simulink model "Galvo_sys_v1"  (R2013a)
settings: Solver=ode45  StartTime=0.0  StopTime=SimEnd  MaxStep=1e-7  RelTol=1e-3
PreLoadFcn:
  | SimEnd = evalin('base','SimEnd');
  | Kp_cc = evalin('base',paramCtrl.Kp_cc);
  | CC_EN = 1;
  | Kp_ccMod = Kp_cc;
InitFcn:
  | Kp_cc=evalin('base',paramCtrl.Kp_cc);
  | 
  | %an = getCallbackAnnotation;
  | %switch CC_EN
  |  %  case 1
  | %        an.Text='Current controller OFF';
  |  %       CC_EN = 0;
  |  %       Kp_ccMod = 1;
  | %      set_param('Galvo_sys_v1/EN_cc','Commented','on')
  | %   case 0
  | %        an.Text='Current controller ON';
  | %        CC_EN = 1;
  | %     set_param('Galvo_sys_v1/EN_cc','Commented','off')
  | %end
  | Kp_ccMod = Kp_cc*CC_EN;
model workspace (MATLAB code in the model file):
  | CC_EN=1;
libraries: simulink x2
settings Model: BufferReuse=off  Creator=mainster  LastModifiedBy=mainster
settings OptimizationCC: InlineParams=on  BufferReuse=off
settings DebuggingCC: SolverPrmCheckMsg=none  InitInArrayFormatMsg=none
settings ModelReferenceCC: ModelReferenceNumInstancesAllowed=Single  ModelReferenceMinAlgLoopOccurrences=on

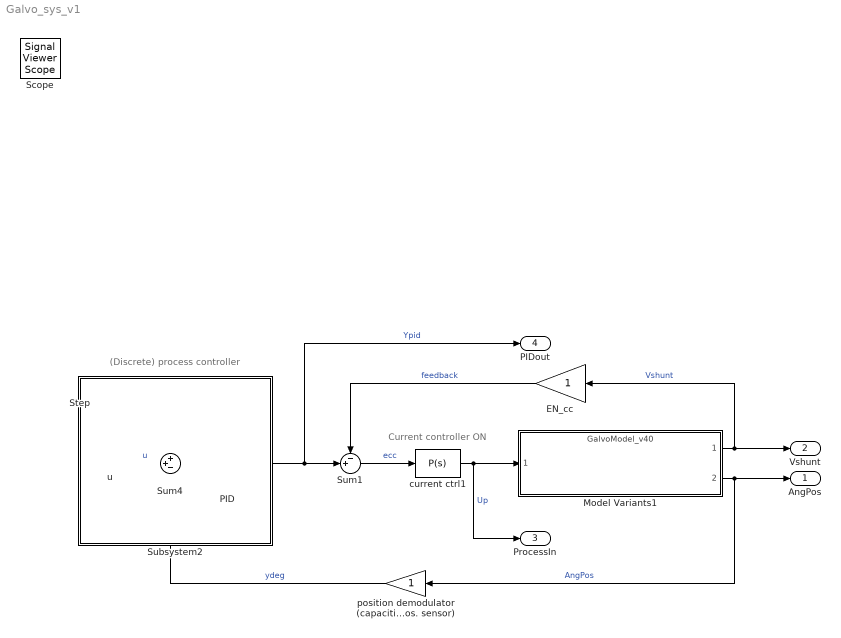
== system Galvo_sys_v1 ==
  note: (Discrete) process controller
  note: Current controller ON
  u : Inport
  EN_cc : Gain
  Model Variants1 : ModelReference  ModelNameDialog=GalvoModel_v40.slx  SimulationMode=Normal  Variant=on  OverrideUsingVariant=Galvo_v40  ModelReferenceVersion=1.24  CopyOfModelName=GalvoModel_v40.slx  DefaultDataLogging=on  mask{modVers=v4.0}
      mask prompts: modVers "Galvo Model version"
      mask init:
      | % switch modVers
      | %     case 'v3.1'
      | %        
      | evalin('base', ['param=loadGalvoParam(' strrep(modVers(2:end-1),'.','') ')'])
      | 
      | switch modVers(1:2)
      |     case 'v4'
      |                 JR=evalin('base','param.JR');
      |                 KMT=evalin('base','param.KMT');
      |                 Rc=evalin('base','param.Rc');
      |                 Lc=evalin('base','param.Lc');
      |                 KFR=evalin('base','param.KFR');
      |                 KTB=evalin('base','param.KTB');
      |                 KBM=evalin('base','param.KBM');
      |                 Rsh=evalin('base','param.Rsh');
      |     case 'v3'
      | 
      |                 RIN=evalin('base','param.RIN');
      |                 TRC=evalin('base','param.TRC');
      |                 CR=evalin('base','param.CR');
      |                 CL=evalin('base','param.CL');
      |                 FR=evalin('base','param.FR');
      |                 KTR=evalin('base','param.KTR');
      |                 BEM=evalin('base','param.BEM');
      |                 SHR=evalin('base','param.SHR');
      |     otherwise
      | 
      | end
      | 
      | set_param(gcb, 'OverrideUsingVariant',sprintf('Galvo_%s',strrep(modVers,'.','')))
      settings: AttributesFormatString=%<ActiveVariant>
      mask TypeOptions modVers: v3.1 | v4.0
      mask Display:
      | str=sprintf('%s',get(gcbh,'ModelName'));
      | port_label('input', 1, 'VCoil','texmode','on')
      | color('blue');
      | port_label('output', 1, 'VShunt','texmode','on')
      | color('black');
      | port_label('output', 2, 'AngPos')
      | %text(.05,.98,['{\fontsize{12}\it\bf' strrep(str,'_',' ') '}'],'horizontalAlignment','left','verticalAlignment','top','texmode','on')
      | text(.015,.98,['{\fontsize{12}\it\bf' strrep(str,'_','\_') '}'],'horizontalAlignment','left','verticalAlignment','top','texmode','on')
  PID : simulink/Continuous/PID Controller  Controller=PID  TimeDomain=Continuous-time  SampleTime=1  IntegratorMethod=Forward Euler  FilterMethod=Forward Euler  Form=Ideal  P=0.0138758158366019  I=3.74215153151693  D=0.0243967322556345  N=1011.12685306507  InitialConditionSource=internal  InitialConditionForIntegrator=0  InitialConditionForFilter=0  ExternalReset=none  IgnoreLimit=on  LimitOutput=on  UpperSaturationLimit=2.5  LowerSaturationLimit=-2.5  LinearizeAsGain=on  AntiWindupMode=back-calculation  Kb=0.8  TrackingMode=off  Kt=0  PParamMin=[]  PParamMax=[]  IParamMin=[]  IParamMax=[]  DParamMin=[]  DParamMax=[]  NParamMin=[]  NParamMax=[]  KbParamMin=[]  KbParamMax=[]  KtParamMin=[]  KtParamMax=[]  POutMin=[]  POutMax=[]  IOutMin=[]  IOutMax=[]  DOutMin=[]  DOutMax=[]  NOutMin=[]  NOutMax=[]  KbOutMin=[]  KbOutMax=[]  KtOutMin=[]  KtOutMax=[]  IntegratorOutMin=[]  IntegratorOutMax=[]  FilterOutMin=[]  FilterOutMax=[]  SumOutMin=[]  SumOutMax=[]  SumI1OutMin=[]  SumI1OutMax=[]  SumI2OutMin=[]  SumI2OutMax=[]  SumI3OutMin=[]  SumI3OutMax=[]  SumDOutMin=[]  SumDOutMax=[]  SaturationOutMin=[]  SaturationOutMax=[]  IntegratorContinuousStateAttributes=''  IntegratorStateMustResolveToSignalObject=off  IntegratorRTWStateStorageClass=Auto  FilterContinuousStateAttributes=''  FilterStateMustResolveToSignalObject=off  FilterRTWStateStorageClass=Auto
  Step : Step  Time=1e-3  SampleTime=0  ZeroCross=off
      settings: AttributesFormatString=Ampl.: %<After>
  Subsystem2 : Subsystem  mask{d=0}
      mask Display: disp('')
  Sum1 : Sum  Inputs=-+|
  Sum4 : Sum  Inputs=++-
  current ctrl1 : simulink/Continuous/PID Controller  Controller=P  TimeDomain=Continuous-time  SampleTime=1  IntegratorMethod=Forward Euler  FilterMethod=Forward Euler  Form=Parallel  P=Kp_ccMod  I=0.7525  D=0.156  N=100  InitialConditionSource=internal  InitialConditionForIntegrator=0  InitialConditionForFilter=0  ExternalReset=none  LimitOutput=on  UpperSaturationLimit=25  LowerSaturationLimit=-25  LinearizeAsGain=on  AntiWindupMode=none  Kb=1  TrackingMode=off  Kt=1  PParamMin=[]  PParamMax=[]  IParamMin=[]  IParamMax=[]  DParamMin=[]  DParamMax=[]  NParamMin=[]  NParamMax=[]  KbParamMin=[]  KbParamMax=[]  KtParamMin=[]  KtParamMax=[]  POutMin=[]  POutMax=[]  IOutMin=[]  IOutMax=[]  DOutMin=[]  DOutMax=[]  NOutMin=[]  NOutMax=[]  KbOutMin=[]  KbOutMax=[]  KtOutMin=[]  KtOutMax=[]  IntegratorOutMin=[]  IntegratorOutMax=[]  FilterOutMin=[]  FilterOutMax=[]  SumOutMin=[]  SumOutMax=[]  SumI1OutMin=[]  SumI1OutMax=[]  SumI2OutMin=[]  SumI2OutMax=[]  SumI3OutMin=[]  SumI3OutMax=[]  SumDOutMin=[]  SumDOutMax=[]  SaturationOutMin=[]  SaturationOutMax=[]  IntegratorContinuousStateAttributes=''  IntegratorStateMustResolveToSignalObject=off  IntegratorRTWStateStorageClass=Auto  FilterContinuousStateAttributes=''  FilterStateMustResolveToSignalObject=off  FilterRTWStateStorageClass=Auto
  position demodulator (capacitive angular pos. sensor) : Gain
  AngPos : Outport
  Vshunt : Outport  Port=2
  ProcessIn : Outport  Port=3
  PIDout : Outport  Port=4
  Scope : SignalViewerScope  IOType=viewer  NumInputPorts=4  LegendLocations=|  RefreshTime=0.038218
      | 0.84205     0.92989     0.11987    0.023866
      | 0.84205     0.69481     0.11987    0.023866
      | 0.87384     0.45973    0.088079    0.023866
      | 0.85795     0.22584     0.10397    0.023866
      settings: ShowLegends=on  TimeRange=0.03  YMin=-0.075~-0.1~-2.5~-0.1  YMax=0.35~1.2~25~0.4
  wires:
  Sum4/1 -> PID/1
  Step/1 -> Sum4/1
  u/1 -> Sum4/2  "u"
  position demodulator (capacitive angular pos. sensor)/1 -> Sum4/3  "ydeg"
  Sum1/1 -> current ctrl1/1  "ecc"
  Model Variants1/1 -> Vshunt/1, EN_cc/1  "Vshunt"
  current ctrl1/1 -> ProcessIn/1, Model Variants1/1  "Up"
  PID/1 -> PIDout/1, Sum1/2  "Ypid"
  Model Variants1/2 -> AngPos/1, position demodulator (capacitive angular pos. sensor)/1  "AngPos"
  EN_cc/1 -> Sum1/1  "feedback"

== system Galvo_sys_v1/Subsystem2 ==
